simulink model "Wrist_Force_Control_v1_2"  (R2020a)
settings: Solver=ode4  StartTime=0.0  StopTime=inf  FixedStep=0.004  RelTol=1e-3  EnableMultiTasking=on
libraries: xpcethercatlib x17, slrtlib x12, simulink x4, simulink_extras x2
settings Model: xpc_rtwmakecfg_data=_xpcethercatlib_  SimulationMode=external  Creator=Ali  LastModifiedBy=Ali
settings SolverCC: ConcurrentTasks=on  AutoInsertRateTranBlk=on
settings DataIOCC: SaveFormat=StructureWithTime
settings OptimizationCC: BlockReduction=off  OptimizeBlockIOStorage=off
settings HardwareCC: ProdBitPerPointer=32  ProdBitPerSizeT=32  ProdBitPerPtrDiffT=32  ProdLargestAtomicFloat=None  ProdWordSize=32  ProdLongLongMode=on  ProdHWDeviceType=Generic->32-bit x86 compatible
settings RTWCC: Description=Simulink Real-Time  SystemTargetFile=slrt.tlc  TemplateMakefile=slrt_default_tmf  CodeExecutionProfiling=on  RTWCompilerOptimization=on
settings SimulinkRealTimeCC: SupportVariableSizeSignals=on  RL32LogTETModifier=off  xPCConcurrentTasks=on

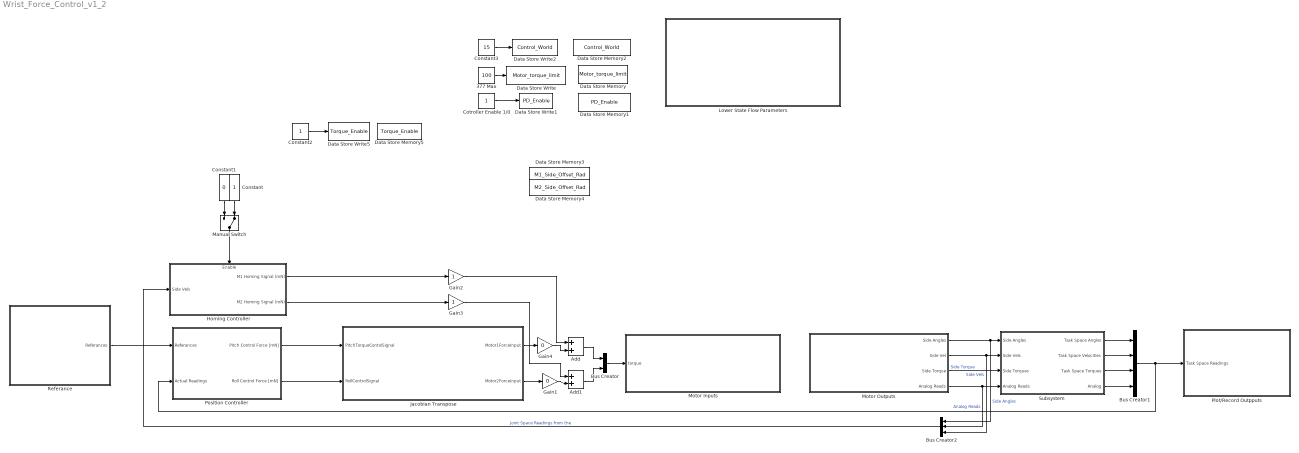
== system Wrist_Force_Control_v1_2 ==
  377 Max : Constant  Value=100
  Add : Sum
  Add1 : Sum
  Bus Creator : BusCreator  Inputs=2
  Bus Creator1 : BusCreator  Inputs=4
  Bus Creator2 : BusCreator  Inputs=3
  Constant : Constant
  Constant1 : Constant  Value=0
  Constant2 : Constant
  Constant3 : Constant  Value=15
  Cotroller Enable 1/0 : Constant
  Data Store Memory : DataStoreMemory  DataStoreName=Motor_torque_limit  ReadBeforeWriteMsg=warning  WriteAfterWriteMsg=warning  WriteAfterReadMsg=warning  ShowAdditionalParam=off
  Data Store Memory1 : DataStoreMemory  DataStoreName=PD_Enable  ReadBeforeWriteMsg=warning  WriteAfterWriteMsg=warning  WriteAfterReadMsg=warning  ShowAdditionalParam=off
  Data Store Memory2 : DataStoreMemory  DataStoreName=Control_World  ReadBeforeWriteMsg=warning  WriteAfterWriteMsg=warning  WriteAfterReadMsg=warning  ShowAdditionalParam=off
  Data Store Memory3 : DataStoreMemory  DataStoreName=M1_Side_Offset_Rad  ReadBeforeWriteMsg=warning  WriteAfterWriteMsg=warning  WriteAfterReadMsg=warning  ShowAdditionalParam=off
  Data Store Memory4 : DataStoreMemory  DataStoreName=M2_Side_Offset_Rad  ReadBeforeWriteMsg=warning  WriteAfterWriteMsg=warning  WriteAfterReadMsg=warning  ShowAdditionalParam=off
  Data Store Memory5 : DataStoreMemory  DataStoreName=Torque_Enable  ReadBeforeWriteMsg=warning  WriteAfterWriteMsg=warning  WriteAfterReadMsg=warning  ShowAdditionalParam=off
  Data Store Write : DataStoreWrite  DataStoreName=Motor_torque_limit
  Data Store Write1 : DataStoreWrite  DataStoreName=PD_Enable
  Data Store Write2 : DataStoreWrite  DataStoreName=Control_World
  Data Store Write5 : DataStoreWrite  DataStoreName=Torque_Enable
  Gain1 : Gain  Gain=0
  Gain2 : Gain
  Gain3 : Gain
  Gain4 : Gain  Gain=0
  Homing Controller : Subsystem
      settings: PortSchema="{\"entries\":[{\"content\":{\"sides\":[{\"content\":{\"connectorIds\":[\"In1\"]},\"type\":\"ConnectorPlacement.EquallySpacedRectSide\",\"uuid\":\"26584363-ec53-497c-894b-995f7264c9bf\"},{\"content\":{\"connectorIds\":[\"Out1\",\"Out2\"],\"side\":\"RIGHT\"},\"type\":\"ConnectorPlacement.EquallySpacedRectSide\",\"uuid\":\"844e0c8d-cb22-473f-a9ac-689e1ce20542\"},{\"content\":{\"connectorIds\":[\"In2\"],\"side\":\"TOP\"},\"type\":\"ConnectorPlacement.EquallySpacedRectSide\",\"uuid\":\"deb693f2-d5e7-4749-a5a4-0b0846583d72\"}]},\"type\":\"ConnectorPlacement.EquallySpacedConnector\",\"uuid\":\"b5658ea7-d246-475e-8f63-4337504fb7e8\"}],\"packageUris\":[\"http://schema.mathworks.com/mf0/Connector/19700101\"],\"version\":\"1.0\"}"
  Jacobian Transpose : MATLAB Function  TreatAsAtomicUnit=on
  Lower State Flow Parameters : Subsystem
  Manual Switch : ManualSwitch  CurrentSetting=0
  Motor Inputs : Subsystem
  Motor Outputs : Subsystem
  Plot/Record Outpputs : Subsystem
  Position Controller : Subsystem
  Referance : Subsystem
  Subsystem : Subsystem
  wires:
  Constant3/1 -> Data Store Write2/1
  377 Max/1 -> Data Store Write/1
  Bus Creator/1 -> Motor Inputs/1(torque)
  Motor Outputs/1(Side Angles) -> Bus Creator2/1, Subsystem/1(Side Angles)  "Side Angles"
  Motor Outputs/2(Side Vel) -> Bus Creator2/3, Subsystem/2(Side Vels)  "Side Vels"
  Motor Outputs/3(Side Torque) -> Subsystem/3(Side Torques)  "Side Torque"
  Motor Outputs/4(Analog Reads) -> Bus Creator2/2, Subsystem/4(Analog Reads)  "Analog Reads"
  Subsystem/1(Task Space Angles) -> Bus Creator1/1
  Subsystem/2(Task Space Velocities) -> Bus Creator1/2
  Subsystem/3(Task Space Torques) -> Bus Creator1/3
  Subsystem/4(Analog) -> Bus Creator1/4
  Bus Creator1/1 -> Position Controller/2(Actual Readings), Plot/Record Outpputs/1(Task Space Readings)
  Referance/1(Referances) -> Position Controller/1(Referances)
  Cotroller Enable 1/0/1 -> Data Store Write1/1
  Position Controller/1(Pitch Control Force [mN]) -> Jacobian Transpose/1(PitchTorqueContolSignal)
  Position Controller/2(Roll Control Force [mN]) -> Jacobian Transpose/2(RollControlSignal)
  Jacobian Transpose/1(Motor1ForceInput) -> Gain4/1
  Add/1 -> Bus Creator/1
  Jacobian Transpose/2(Motor2ForceInput) -> Gain1/1
  Add1/1 -> Bus Creator/2
  Constant/1 -> Manual Switch/2
  Constant1/1 -> Manual Switch/1
  Constant2/1 -> Data Store Write5/1
  Gain4/1 -> Add/2
  Gain1/1 -> Add1/2
  Gain2/1 -> Add/1
  Gain3/1 -> Add1/1
  Manual Switch/1 -> Homing Controller/2(Enable)
  Homing Controller/1(M1 Homing Signal (mN)) -> Gain2/1
  Homing Controller/2(M2 Homing Signal (mN)) -> Gain3/1
  Bus Creator2/1 -> Homing Controller/1(Side Vels)  "Joint Space Readings from the"

== system Wrist_Force_Control_v1_2/Homing Controller ==
  Side Vels : Inport
  Enable : Inport  Port=2
  Analog Homing Controllers : Subsystem
  Bus Selector : BusSelector  OutputSignals=Analog Reads,Side Vels,Side Angles
  Clock : Subsystem
  M1 Homing Signal (mN) : Outport
  M2 Homing Signal (mN) : Outport  Port=2
  wires:
  Analog Homing Controllers/1(M1 Homing Signal) -> M1 Homing Signal (mN)/1  "M1 Homing Signal (mN)"
  Clock/1(Enabling Signal) -> Analog Homing Controllers/Enable
  Enable/1 -> Clock/Enable
  Analog Homing Controllers/2(M2 Homing Signal) -> M2 Homing Signal (mN)/1  "M2 Homing Signal (mN)"
  Side Vels/1 -> Bus Selector/1
  Bus Selector/1 -> Analog Homing Controllers/1(Analog Signals)  "<Analog Reads>"
  Bus Selector/2 -> Analog Homing Controllers/2(Side Vels)  "<Side Vels>"
  Bus Selector/3 -> Analog Homing Controllers/3(Side Angles)  "<Side Angles>"

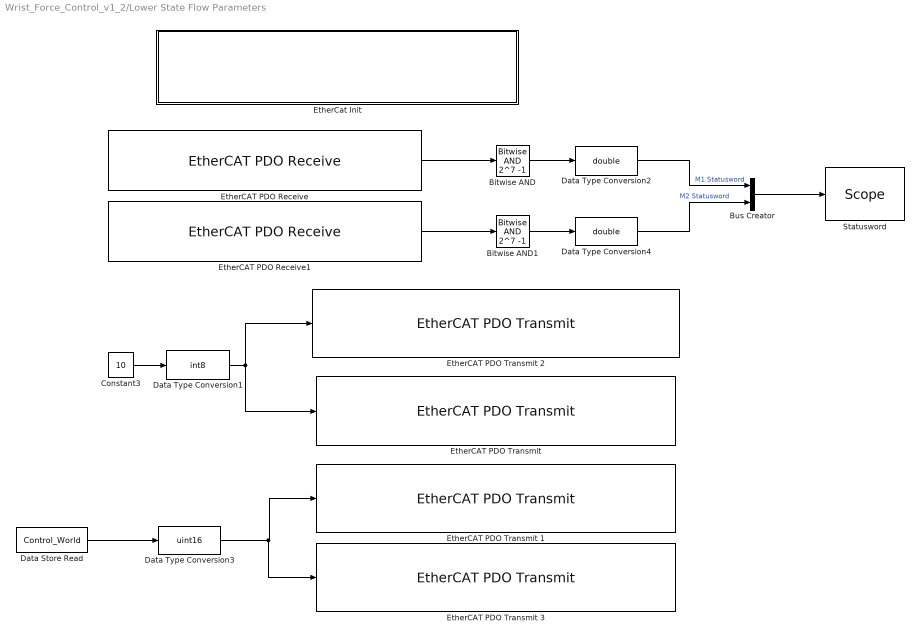
== system Wrist_Force_Control_v1_2/Lower State Flow Parameters ==
  Bitwise AND : simulink/Logic and Bit Operations/Bitwise Operator  logicop=AND  UseBitMask=on  BitMask=2^7 -1  BitMaskRealWorld=Stored Integer
  Bitwise AND1 : simulink/Logic and Bit Operations/Bitwise Operator  logicop=AND  UseBitMask=on  BitMask=2^7 -1  BitMaskRealWorld=Stored Integer
  Bus Creator : BusCreator  Inputs=2
  Constant3 : Constant  Value=10
  Data Store Read : DataStoreRead  DataStoreName=Control_World
  Data Type Conversion1 : DataTypeConversion  OutDataTypeStr=int8
  Data Type Conversion2 : DataTypeConversion  OutDataTypeStr=double
  Data Type Conversion3 : DataTypeConversion  OutDataTypeStr=uint16
  Data Type Conversion4 : DataTypeConversion  OutDataTypeStr=double
  EtherCAT PDO Receive : xpcethercatlib/EtherCAT PDO Receive  Priority=2  sig_name=M1.Module 1 (CST Mode).CST Inputs.Statusword  sig_offset=568  sig_type=uint16  type_size=16  sig_dim=1  device_id=0  sample_time=0.004000
      settings: SourceProductBaseCode=XP
  EtherCAT PDO Receive1 : xpcethercatlib/EtherCAT PDO Receive  Priority=2  sig_name=M2.Module 1 (CST Mode).CST Inputs.Statusword  sig_offset=696  sig_type=uint16  type_size=16  sig_dim=1  device_id=0  sample_time=0.004000
      settings: SourceProductBaseCode=XP
  "EtherCAT PDO Transmit " : xpcethercatlib/EtherCAT PDO Transmit   Priority=3  sig_name=M2.Module 1 (CST Mode).CST Outputs.Mode of operation  sig_offset=728  sig_type=int8  type_size=8  sig_dim=1  device_id=0  sample_time=0.004000
      settings: SourceProductBaseCode=XP
  EtherCAT PDO Transmit 1 : xpcethercatlib/EtherCAT PDO Transmit   Priority=3  sig_name=M1.Module 1 (CST Mode).CST Outputs.Controlword  sig_offset=568  sig_type=uint16  type_size=16  sig_dim=1  device_id=0  sample_time=0.004000
      settings: SourceProductBaseCode=XP
  EtherCAT PDO Transmit 2 : xpcethercatlib/EtherCAT PDO Transmit   Priority=3  sig_name=M1.Module 1 (CST Mode).CST Outputs.Mode of operation  sig_offset=600  sig_type=int8  type_size=8  sig_dim=1  device_id=0  sample_time=0.004000
      settings: SourceProductBaseCode=XP
  EtherCAT PDO Transmit 3 : xpcethercatlib/EtherCAT PDO Transmit   Priority=3  sig_name=M2.Module 1 (CST Mode).CST Outputs.Controlword  sig_offset=696  sig_type=uint16  type_size=16  sig_dim=1  device_id=0  sample_time=0.004000
      settings: SourceProductBaseCode=XP
  EtherCat Init : Subsystem
  Statusword : slrtlib/Displays and Logging/Scope   scopeno=1  scopetype=Target  autostart=on  viewmode=Numerical  formatstr='%15.6f'  grid=on  ylimits=[0,0]  nosamples=100  noprepostsamples=0  interleave=5  triggermode=FreeRun  triggersignal=1  trigsignalfromport=off  triggerlevel=0.0  triggerslope=Either  triggerscope=1  triggersample=0  filename=data.dat  mode=Lazy  writesize=512  autorestart=off  dynamicfilemode=off  maxwritefilesize=512*1024^2
  wires:
  Bitwise AND/1 -> Data Type Conversion2/1
  EtherCAT PDO Receive/1 -> Bitwise AND/1
  Data Store Read/1 -> Data Type Conversion3/1
  Constant3/1 -> Data Type Conversion1/1
  Data Type Conversion1/1 -> EtherCAT PDO Transmit 2/1, "EtherCAT PDO Transmit "/1
  Bitwise AND1/1 -> Data Type Conversion4/1
  EtherCAT PDO Receive1/1 -> Bitwise AND1/1
  Data Type Conversion4/1 -> Bus Creator/2  "M2 Statusword"
  Bus Creator/1 -> Statusword/1
  Data Type Conversion2/1 -> Bus Creator/1  "M1 Statusword"
  Data Type Conversion3/1 -> EtherCAT PDO Transmit 3/1, EtherCAT PDO Transmit 1/1

== system Wrist_Force_Control_v1_2/Motor Inputs ==
  torque : Inport
  "M1 Target Torque " : xpcethercatlib/EtherCAT PDO Transmit   Priority=3  sig_name=M1.Module 1 (CST Mode).CST Outputs.Target torque  sig_offset=584  sig_type=int16  type_size=16  sig_dim=1  device_id=0  sample_time=0.004000
      settings: SourceProductBaseCode=XP
  M2 Target Torque : xpcethercatlib/EtherCAT PDO Transmit   Priority=3  sig_name=M2.Module 1 (CST Mode).CST Outputs.Target torque  sig_offset=712  sig_type=int16  type_size=16  sig_dim=1  device_id=0  sample_time=0.004000
      settings: SourceProductBaseCode=XP
  "Scope " : slrtlib/Displays and Logging/Scope   Commented=on  scopeno=2  scopetype=Target  autostart=on  viewmode=Graphical rolling  formatstr='%15.6f'  grid=on  ylimits=[0,0]  nosamples=100  noprepostsamples=0  interleave=5  triggermode=FreeRun  triggersignal=1  trigsignalfromport=off  triggerlevel=0.0  triggerslope=Either  triggerscope=1  triggersample=0  filename=data.dat  mode=Lazy  writesize=512  autorestart=off  dynamicfilemode=off  maxwritefilesize=512*1024^2
  "Torque Mappig and Saturation " : Subsystem
  wires:
  torque/1 -> "Torque Mappig and Saturation "/1(torque)
  "Torque Mappig and Saturation "/3(Motor Torques) -> "Scope "/1
  "Torque Mappig and Saturation "/1(M1_torque) -> "M1 Target Torque "/1
  "Torque Mappig and Saturation "/2(M2_torque) -> M2 Target Torque/1

== system Wrist_Force_Control_v1_2/Motor Outputs ==
  Analog Readigs : Subsystem
  Angle Readigs : Subsystem
  Bus Creator : BusCreator  Inputs=2
  Torque Readings : Subsystem
  Velocity Readings : Subsystem
  Side Angles : Outport
  Side Vel : Outport  Port=2
  Side Torque : Outport  Port=3
  Analog Reads : Outport  Port=4
  wires:
  Velocity Readings/1(Side Vel) -> Side Vel/1
  Torque Readings/1(Side Torque) -> Side Torque/1
  Angle Readigs/1(Side angles) -> Side Angles/1
  Analog Readigs/1(M1 Analog Reads (mV)) -> Bus Creator/1  "M1 Analog Reads"
  Analog Readigs/2(M2 Analog Reads (mV)) -> Bus Creator/2  "M2 Analog Reads"
  Bus Creator/1 -> Analog Reads/1

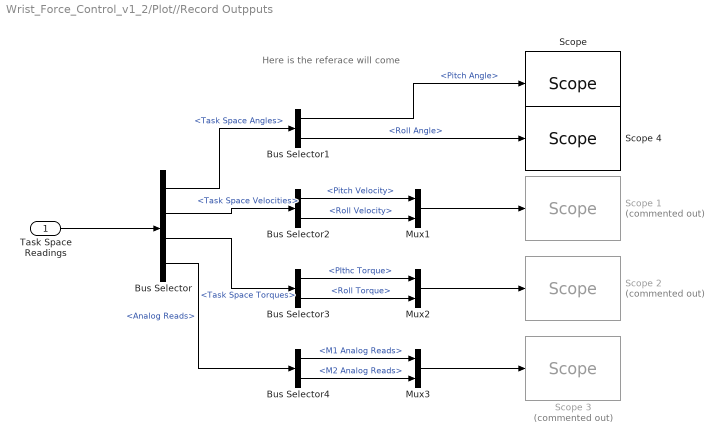
== system Wrist_Force_Control_v1_2/Plot//Record Outpputs ==
  note: Here is the referace will come
  Task Space Readings : Inport
  Bus Selector : BusSelector  OutputSignals=Task Space Angles,Task Space Velocities,Task Space Torques,Analog Reads
  Bus Selector1 : BusSelector  OutputSignals=Pitch Angle,Roll Angle
  Bus Selector2 : BusSelector  OutputSignals=Pitch Velocity,Roll Velocity
  Bus Selector3 : BusSelector  OutputSignals=PIthc Torque,Roll Torque
  Bus Selector4 : BusSelector  OutputSignals=M1 Analog Reads,M2 Analog Reads
  Mux1 : Mux  Inputs=2
  Mux2 : Mux  Inputs=2
  Mux3 : Mux  Inputs=2
  "Scope " : slrtlib/Displays and Logging/Scope   scopeno=8  scopetype=Target  autostart=on  viewmode=Graphical rolling  formatstr='%15.6f'  grid=on  ylimits=[0,0]  nosamples=100  noprepostsamples=0  interleave=5  triggermode=FreeRun  triggersignal=1  trigsignalfromport=off  triggerlevel=0.0  triggerslope=Either  triggerscope=1  triggersample=0  filename=data.dat  mode=Lazy  writesize=512  autorestart=off  dynamicfilemode=off  maxwritefilesize=512*1024^2
  Scope 1 : slrtlib/Displays and Logging/Scope   Commented=on  scopeno=4  scopetype=Target  autostart=on  viewmode=Graphical rolling  formatstr='%15.6f'  grid=on  ylimits=[0,0]  nosamples=500  noprepostsamples=0  interleave=20  triggermode=FreeRun  triggersignal=1  trigsignalfromport=off  triggerlevel=0.0  triggerslope=Either  triggerscope=1  triggersample=0  filename=data.dat  mode=Lazy  writesize=512  autorestart=off  dynamicfilemode=off  maxwritefilesize=512*1024^2
  Scope 2 : slrtlib/Displays and Logging/Scope   Commented=on  scopeno=5  scopetype=Target  autostart=on  viewmode=Graphical rolling  formatstr='%15.6f'  grid=on  ylimits=[0,0]  nosamples=500  noprepostsamples=0  interleave=20  triggermode=FreeRun  triggersignal=1  trigsignalfromport=off  triggerlevel=0.0  triggerslope=Either  triggerscope=1  triggersample=0  filename=data.dat  mode=Lazy  writesize=512  autorestart=off  dynamicfilemode=off  maxwritefilesize=512*1024^2
  Scope 3 : slrtlib/Displays and Logging/Scope   Commented=on  scopeno=6  scopetype=Target  autostart=on  viewmode=Graphical rolling  formatstr='%15.6f'  grid=on  ylimits=[0,0]  nosamples=500  noprepostsamples=0  interleave=20  triggermode=FreeRun  triggersignal=1  trigsignalfromport=off  triggerlevel=0.0  triggerslope=Either  triggerscope=1  triggersample=0  filename=data.dat  mode=Lazy  writesize=512  autorestart=off  dynamicfilemode=off  maxwritefilesize=512*1024^2
  Scope 4 : slrtlib/Displays and Logging/Scope   scopeno=9  scopetype=Target  autostart=on  viewmode=Graphical rolling  formatstr='%15.6f'  grid=on  ylimits=[0,0]  nosamples=100  noprepostsamples=0  interleave=5  triggermode=FreeRun  triggersignal=1  trigsignalfromport=off  triggerlevel=0.0  triggerslope=Either  triggerscope=1  triggersample=0  filename=data.dat  mode=Lazy  writesize=512  autorestart=off  dynamicfilemode=off  maxwritefilesize=512*1024^2
  wires:
  Task Space Readings/1 -> Bus Selector/1
  Bus Selector/1 -> Bus Selector1/1  "<Task Space Angles>"
  Bus Selector1/1 -> "Scope "/1  "<Pitch Angle>"
  Bus Selector1/2 -> Scope 4/1  "<Roll Angle>"
  Bus Selector2/1 -> Mux1/1  "<Pitch Velocity>"
  Mux1/1 -> Scope 1/1
  Bus Selector2/2 -> Mux1/2  "<Roll Velocity>"
  Bus Selector/2 -> Bus Selector2/1  "<Task Space Velocities>"
  Bus Selector3/2 -> Mux2/2  "<Roll Torque>"
  Bus Selector3/1 -> Mux2/1  "<PIthc Torque>"
  Mux2/1 -> Scope 2/1
  Bus Selector/3 -> Bus Selector3/1  "<Task Space Torques>"
  Mux3/1 -> Scope 3/1
  Bus Selector4/2 -> Mux3/2  "<M2 Analog Reads>"
  Bus Selector4/1 -> Mux3/1  "<M1 Analog Reads>"
  Bus Selector/4 -> Bus Selector4/1  "<Analog Reads>"

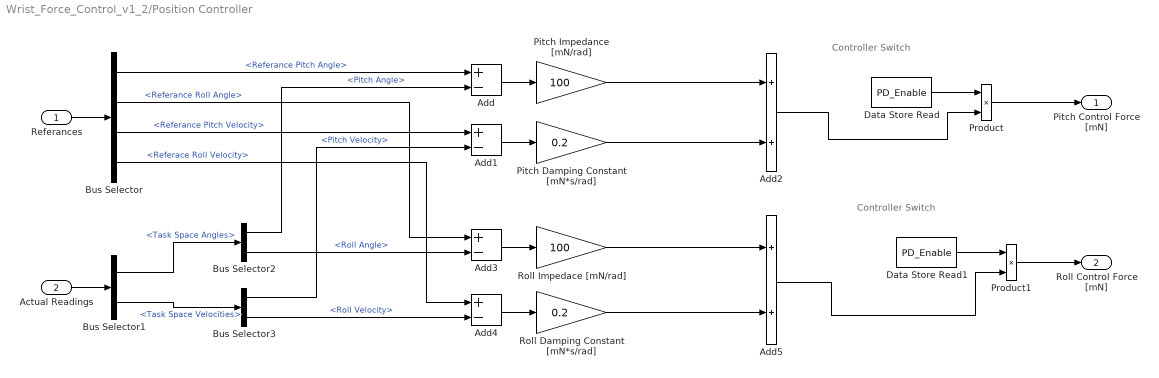
== system Wrist_Force_Control_v1_2/Position Controller ==
  note: Controller Switch
  note: Controller Switch
  Referances : Inport
  Actual Readings : Inport  Port=2
  Add{,1,3..4} (4 alike) : Sum  Inputs=+-
  Add2 : Sum
  Add5 : Sum
  Bus Selector : BusSelector  OutputSignals=Referance Pitch Angle,Referance Roll Angle,Referance Pitch Velocity,Referace Roll Velocity
  Bus Selector1 : BusSelector  OutputSignals=Task Space Angles,Task Space Velocities
  Bus Selector2 : BusSelector  OutputSignals=Pitch Angle,Roll Angle
  Bus Selector3 : BusSelector  OutputSignals=Pitch Velocity,Roll Velocity
  Data Store Read : DataStoreRead  DataStoreName=PD_Enable
  Data Store Read1 : DataStoreRead  DataStoreName=PD_Enable
  Pitch Damping Constant [mN*s/rad] : Gain  Gain=0.2
  Pitch Impedance [mN/rad] : Gain  Gain=100
  Product : Product
  Product1 : Product
  Roll Damping Constant [mN*s/rad] : Gain  Gain=0.2
  Roll Impedace [mN/rad] : Gain  Gain=100
  Pitch Control Force [mN] : Outport
  Roll Control Force [mN] : Outport  Port=2
  wires:
  Referances/1 -> Bus Selector/1
  Bus Selector/1 -> Add/1  "<Referance Pitch Angle>"
  Bus Selector/2 -> Add3/1  "<Referance Roll Angle>"
  Bus Selector/4 -> Add4/1  "<Referace Roll Velocity>"
  Actual Readings/1 -> Bus Selector1/1
  Add/1 -> Pitch Impedance [mN/rad]/1
  Pitch Damping Constant [mN*s/rad]/1 -> Add2/2
  Product/1 -> Pitch Control Force [mN]/1
  Add2/1 -> Product/2
  Data Store Read/1 -> Product/1
  Add1/1 -> Pitch Damping Constant [mN*s/rad]/1
  Bus Selector1/1 -> Bus Selector2/1  "<Task Space Angles>"
  Bus Selector1/2 -> Bus Selector3/1  "<Task Space Velocities>"
  Bus Selector2/1 -> Add/2  "<Pitch Angle>"
  Bus Selector/3 -> Add1/1  "<Referance Pitch Velocity>"
  Bus Selector3/1 -> Add1/2  "<Pitch Velocity>"
  Bus Selector3/2 -> Add4/2  "<Roll Velocity>"
  Bus Selector2/2 -> Add3/2  "<Roll Angle>"
  Add3/1 -> Roll Impedace [mN/rad]/1
  Add4/1 -> Roll Damping Constant [mN*s/rad]/1
  Pitch Impedance [mN/rad]/1 -> Add2/1
  Roll Impedace [mN/rad]/1 -> Add5/1
  Roll Damping Constant [mN*s/rad]/1 -> Add5/2
  Product1/1 -> Roll Control Force [mN]/1
  Add5/1 -> Product1/2
  Data Store Read1/1 -> Product1/1

== system Wrist_Force_Control_v1_2/Referance ==
  Bus Creator : BusCreator  Inputs=4
  Degrees to Radians : simulink_extras/Transformations/Degrees to Radians
  Degrees to Radians1 : simulink_extras/Transformations/Degrees to Radians
  Pitch Degree : Constant
  Pitch Velocity (rad/s) : Constant
  Roll Degree : Constant
  Roll Velocity (rad/s) : Constant
  Referances : Outport
  wires:
  Pitch Degree/1 -> Degrees to Radians/1
  Roll Degree/1 -> Degrees to Radians1/1
  Degrees to Radians1/1 -> Bus Creator/2  "Referance Roll Angle"
  Pitch Velocity (rad/s)/1 -> Bus Creator/3  "Referance Pitch Velocity"
  Roll Velocity (rad/s)/1 -> Bus Creator/4  "Referace Roll Velocity"
  Degrees to Radians/1 -> Bus Creator/1  "Referance Pitch Angle"
  Bus Creator/1 -> Referances/1

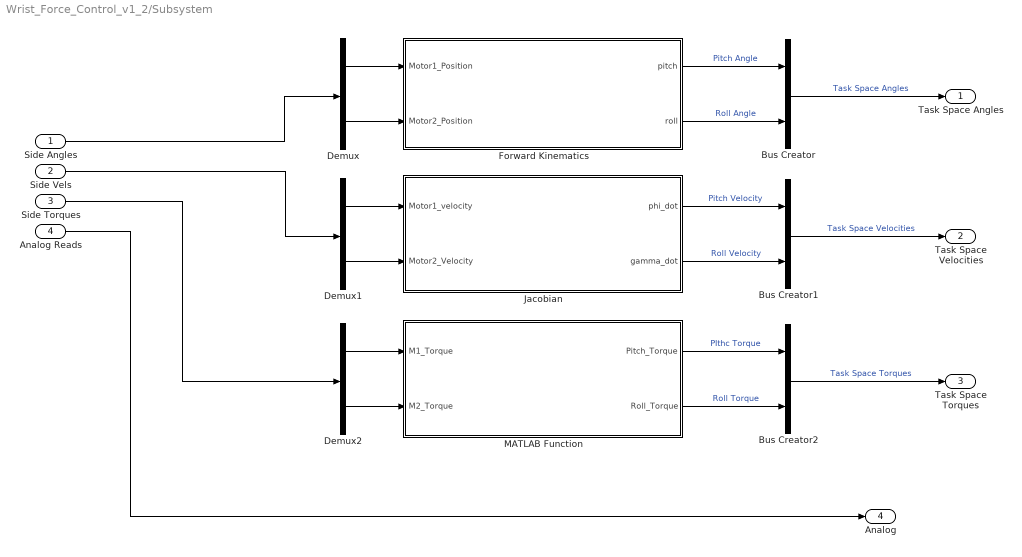
== system Wrist_Force_Control_v1_2/Subsystem ==
  Side Angles : Inport
  Side Vels : Inport  Port=2
  Side Torques : Inport  Port=3
  Analog Reads : Inport  Port=4
  Bus Creator : BusCreator  Inputs=2
  Bus Creator1 : BusCreator  Inputs=2
  Bus Creator2 : BusCreator  Inputs=2
  Demux : Demux  Outputs=2
  Demux1 : Demux  Outputs=2
  Demux2 : Demux  Outputs=2
  Forward Kinematics : MATLAB Function  TreatAsAtomicUnit=on
  Jacobian : MATLAB Function  TreatAsAtomicUnit=on
  MATLAB Function : MATLAB Function  TreatAsAtomicUnit=on
  Task Space Angles : Outport
  Task Space Velocities : Outport  Port=2
  Task Space Torques : Outport  Port=3
  Analog : Outport  Port=4
  wires:
  Analog Reads/1 -> Analog/1
  Side Torques/1 -> Demux2/1
  Side Angles/1 -> Demux/1
  Demux/1 -> Forward Kinematics/1(Motor1_Position)
  Demux/2 -> Forward Kinematics/2(Motor2_Position)
  Demux1/2 -> Jacobian/2(Motor2_Velocity)
  Demux1/1 -> Jacobian/1(Motor1_velocity)
  Side Vels/1 -> Demux1/1
  Jacobian/1(phi_dot) -> Bus Creator1/1  "Pitch Velocity"
  Jacobian/2(gamma_dot) -> Bus Creator1/2  "Roll Velocity"
  Demux2/1 -> MATLAB Function/1(M1_Torque)
  Demux2/2 -> MATLAB Function/2(M2_Torque)
  Forward Kinematics/1(pitch) -> Bus Creator/1  "Pitch Angle"
  Forward Kinematics/2(roll) -> Bus Creator/2  "Roll Angle"
  Bus Creator/1 -> Task Space Angles/1  "Task Space Angles"
  MATLAB Function/1(Pitch_Torque) -> Bus Creator2/1  "PIthc Torque"
  MATLAB Function/2(Roll_Torque) -> Bus Creator2/2  "Roll Torque"
  Bus Creator2/1 -> Task Space Torques/1  "Task Space Torques"
  Bus Creator1/1 -> Task Space Velocities/1  "Task Space Velocities"

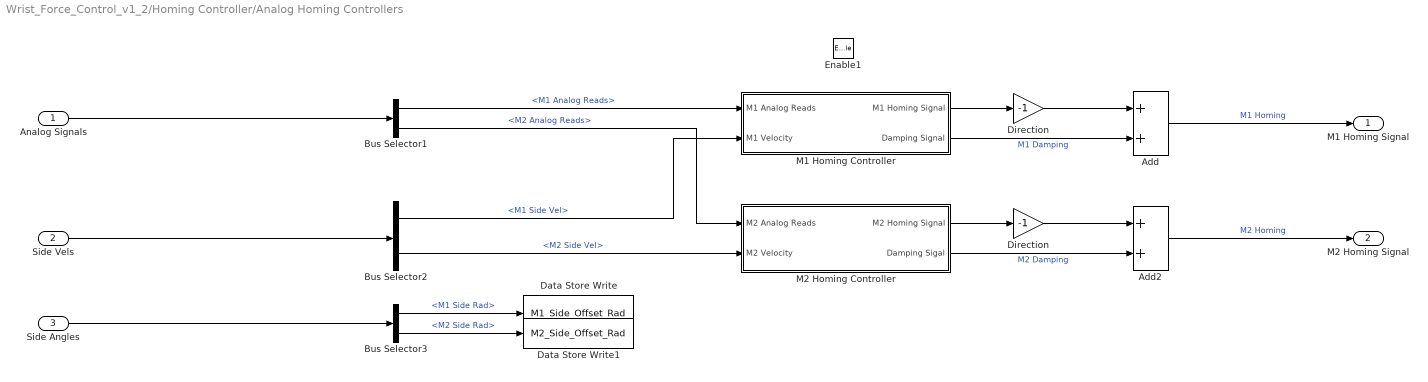
== system Wrist_Force_Control_v1_2/Homing Controller/Analog Homing Controllers ==
  Analog Signals : Inport
  Side Vels : Inport  Port=2
  Side Angles : Inport  Port=3
  Enable1 : EnablePort
  Add : Sum
  Add2 : Sum
  Bus Selector1 : BusSelector  OutputSignals=M1 Analog Reads,M2 Analog Reads
  Bus Selector2 : BusSelector  OutputSignals=M1 Side Vel,M2 Side Vel
  Bus Selector3 : BusSelector  OutputSignals=M1 Side Rad,M2 Side Rad
  Data Store Write : DataStoreWrite  DataStoreName=M1_Side_Offset_Rad
  Data Store Write1 : DataStoreWrite  DataStoreName=M2_Side_Offset_Rad
  Direction : Gain  Gain=-1
  "Direction " : Gain  Gain=-1
  M1 Homing Controller : Subsystem
  M2 Homing Controller : Subsystem
  M1 Homing Signal : Outport
  M2 Homing Signal : Outport  Port=2
  wires:
  Bus Selector1/1 -> M1 Homing Controller/1(M1 Analog Reads)  "<M1 Analog Reads>"
  Analog Signals/1 -> Bus Selector1/1
  Bus Selector1/2 -> M2 Homing Controller/1(M2 Analog Reads)  "<M2 Analog Reads>"
  M1 Homing Controller/1(M1 Homing Signal) -> Direction/1
  M2 Homing Controller/1(M2 Homing Signal) -> "Direction "/1
  Side Vels/1 -> Bus Selector2/1
  Direction/1 -> Add/1
  M1 Homing Controller/2(Damping Signal) -> Add/2  "M1 Damping"
  Add/1 -> M1 Homing Signal/1  "M1 Homing"
  Add2/1 -> M2 Homing Signal/1  "M2 Homing"
  "Direction "/1 -> Add2/1
  M2 Homing Controller/2(Damping Sigal) -> Add2/2  "M2 Damping"
  Bus Selector2/1 -> M1 Homing Controller/2(M1 Velocity)  "<M1 Side Vel>"
  Bus Selector2/2 -> M2 Homing Controller/2(M2 Velocity)  "<M2 Side Vel>"
  Side Angles/1 -> Bus Selector3/1
  Bus Selector3/1 -> Data Store Write/1  "<M1 Side Rad>"
  Bus Selector3/2 -> Data Store Write1/1  "<M2 Side Rad>"

== system Wrist_Force_Control_v1_2/Homing Controller/Clock ==
  Enable : EnablePort
  Clock : Clock
  Constant5 : Constant  Value=10
  Relational Operator : RelationalOperator  OutDataTypeStr=boolean  RndMeth=Simplest
  Enabling Signal : Outport
  wires:
  Clock/1 -> Relational Operator/1
  Constant5/1 -> Relational Operator/2
  Relational Operator/1 -> Enabling Signal/1

== system Wrist_Force_Control_v1_2/Lower State Flow Parameters/EtherCat Init ==
  "EtherCAT Init " : xpcethercatlib/EtherCAT Init   Priority=0  config_file=C:\Users\Ali\Desktop\Wrist_Control_Test\XML_Config_File\Force_Control_v2.5_250Hz.xml  device_id=0  pci_bus=2  pci_slot=0  pci_function=0  initstate=2  dctuning=0  enaDebug=off  enaDC=on  errLink=off  masterDbg=off  stateChgDbg=off  baseClock=off  masterCfg=off  logFile='c:\dbglog.txt'  sample_time=0.004000  DCMode=2
      settings: SourceProductBaseCode=XP
  Terminator : Terminator
  wires:
  "EtherCAT Init "/1 -> Terminator/1

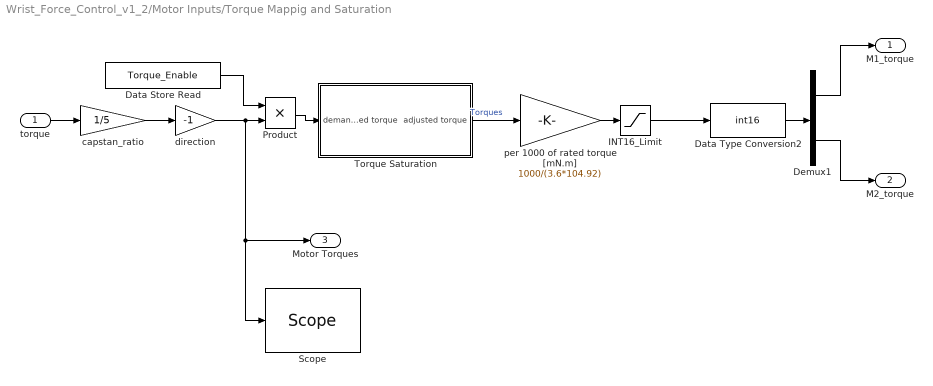
== system Wrist_Force_Control_v1_2/Motor Inputs/Torque Mappig and Saturation  ==
  torque : Inport
  Data Store Read : DataStoreRead  DataStoreName=Torque_Enable
  Data Type Conversion2 : DataTypeConversion  OutDataTypeStr=int16
  Demux1 : Demux  Outputs=2
  INT16_Limit : Saturate  UpperLimit=[2^15-1 2^15-1]  LowerLimit=[-2^15 -2^15]
  Product : Product
  "Scope " : slrtlib/Displays and Logging/Scope   scopeno=5  scopetype=Target  autostart=on  viewmode=Numerical  formatstr='%15.6f'  grid=on  ylimits=[0,0]  nosamples=100  noprepostsamples=0  interleave=5  triggermode=FreeRun  triggersignal=1  trigsignalfromport=off  triggerlevel=0.0  triggerslope=Either  triggerscope=1  triggersample=0  filename=data.dat  mode=Lazy  writesize=512  autorestart=off  dynamicfilemode=off  maxwritefilesize=512*1024^2
  Torque Saturation : Subsystem
  capstan_ratio : Gain  Gain=1/5
  direction : Gain  Gain=-1  OutDataTypeStr=double
  per 1000 of rated torque [mN.m] : Gain  Gain=1000/(3.6*104.92)  OutDataTypeStr=double
  M1_torque : Outport  VectorParamsAs1DForOutWhenUnconnected=off
  M2_torque : Outport  Port=2  VectorParamsAs1DForOutWhenUnconnected=off
  Motor Torques : Outport  Port=3
  wires:
  direction/1 -> Product/2, "Scope "/1, Motor Torques/1
  Demux1/1 -> M1_torque/1
  Demux1/2 -> M2_torque/1
  per 1000 of rated torque [mN.m]/1 -> INT16_Limit/1
  Torque Saturation/1(adjusted torque) -> per 1000 of rated torque [mN.m]/1  "Torques"
  capstan_ratio/1 -> direction/1
  INT16_Limit/1 -> Data Type Conversion2/1
  torque/1 -> capstan_ratio/1
  Data Type Conversion2/1 -> Demux1/1
  Product/1 -> Torque Saturation/1(demanded torque)
  Data Store Read/1 -> Product/1

== system Wrist_Force_Control_v1_2/Motor Outputs/Analog Readigs ==
  Cast To Double : DataTypeConversion  OutDataTypeStr=double
  Cast To Double1 : DataTypeConversion  OutDataTypeStr=double
  EtherCAT PDO Receive : xpcethercatlib/EtherCAT PDO Receive  Priority=2  sig_name=M1.Module 1 (CST Mode).CST Inputs.Analog input general purpose A  sig_offset=680  sig_type=int16  type_size=16  sig_dim=1  device_id=0  sample_time=0.004000
      settings: SourceProductBaseCode=XP
  EtherCAT PDO Receive1 : xpcethercatlib/EtherCAT PDO Receive  Priority=2  sig_name=M2.Module 1 (CST Mode).CST Inputs.Analog input general purpose A  sig_offset=808  sig_type=int16  type_size=16  sig_dim=1  device_id=0  sample_time=0.004000
      settings: SourceProductBaseCode=XP
  Scope 2 : slrtlib/Displays and Logging/Scope   scopeno=3  scopetype=Target  autostart=on  viewmode=Graphical rolling  formatstr='%15.6f'  grid=on  ylimits=[0,0]  nosamples=250  noprepostsamples=0  interleave=5  triggermode=FreeRun  triggersignal=1  trigsignalfromport=off  triggerlevel=0.0  triggerslope=Either  triggerscope=1  triggersample=0  filename=data.dat  mode=Lazy  writesize=512  autorestart=off  dynamicfilemode=off  maxwritefilesize=512*1024^2
  Scope 3 : slrtlib/Displays and Logging/Scope   scopeno=4  scopetype=Target  autostart=on  viewmode=Graphical rolling  formatstr='%15.6f'  grid=on  ylimits=[0,0]  nosamples=250  noprepostsamples=0  interleave=5  triggermode=FreeRun  triggersignal=1  trigsignalfromport=off  triggerlevel=0.0  triggerslope=Either  triggerscope=1  triggersample=0  filename=data.dat  mode=Lazy  writesize=512  autorestart=off  dynamicfilemode=off  maxwritefilesize=512*1024^2
  mV to count : Gain  Gain=1/10
  mV to count1 : Gain  Gain=1/10
  M1 Analog Reads (mV) : Outport
  M2 Analog Reads (mV) : Outport  Port=2
  wires:
  EtherCAT PDO Receive1/1 -> Cast To Double1/1
  EtherCAT PDO Receive/1 -> Cast To Double/1
  Cast To Double/1 -> mV to count1/1  "M1 Analog Read"
  Cast To Double1/1 -> mV to count/1  "M2 Analog Read"
  mV to count1/1 -> Scope 2/1, M1 Analog Reads (mV)/1  "M1 Analog Read"
  mV to count/1 -> Scope 3/1, M2 Analog Reads (mV)/1  "M2 Analog Read"

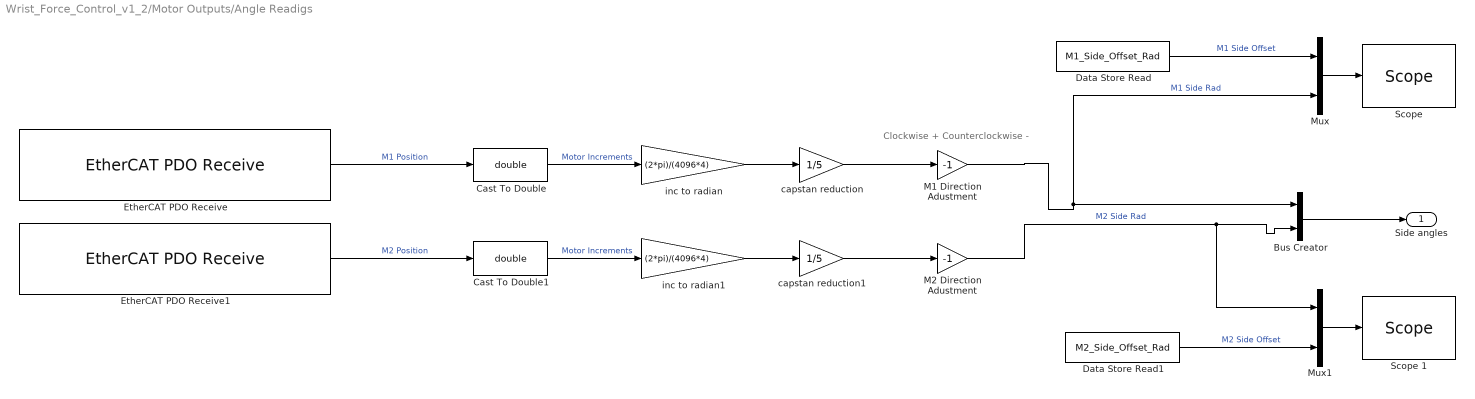
== system Wrist_Force_Control_v1_2/Motor Outputs/Angle Readigs ==
  note: Clockwise + Counterclockwise -
  Bus Creator : BusCreator  Inputs=2
  Cast To Double : DataTypeConversion  OutDataTypeStr=double
  Cast To Double1 : DataTypeConversion  OutDataTypeStr=double
  Data Store Read : DataStoreRead  DataStoreName=M1_Side_Offset_Rad
  Data Store Read1 : DataStoreRead  DataStoreName=M2_Side_Offset_Rad
  EtherCAT PDO Receive : xpcethercatlib/EtherCAT PDO Receive  Priority=2  sig_name=M1.Module 1 (CST Mode).CST Inputs.Position actual value  sig_offset=584  sig_type=int32  type_size=32  sig_dim=1  device_id=0  sample_time=0.004000
      settings: SourceProductBaseCode=XP
  EtherCAT PDO Receive1 : xpcethercatlib/EtherCAT PDO Receive  Priority=2  sig_name=M2.Module 1 (CST Mode).CST Inputs.Position actual value  sig_offset=712  sig_type=int32  type_size=32  sig_dim=1  device_id=0  sample_time=0.004000
      settings: SourceProductBaseCode=XP
  "M1 Direction Adustment " : Gain  Gain=-1
  M2 Direction Adustment : Gain  Gain=-1
  Mux : Mux  Inputs=2
  Mux1 : Mux  Inputs=2
  "Scope " : slrtlib/Displays and Logging/Scope   scopeno=2  scopetype=Target  autostart=on  viewmode=Numerical  formatstr='%15.6f'  grid=on  ylimits=[0,0]  nosamples=100  noprepostsamples=0  interleave=5  triggermode=FreeRun  triggersignal=1  trigsignalfromport=off  triggerlevel=0.0  triggerslope=Either  triggerscope=1  triggersample=0  filename=data.dat  mode=Lazy  writesize=512  autorestart=off  dynamicfilemode=off  maxwritefilesize=512*1024^2
  Scope 1 : slrtlib/Displays and Logging/Scope   scopeno=7  scopetype=Target  autostart=on  viewmode=Numerical  formatstr='%15.6f'  grid=on  ylimits=[0,0]  nosamples=100  noprepostsamples=0  interleave=5  triggermode=FreeRun  triggersignal=1  trigsignalfromport=off  triggerlevel=0.0  triggerslope=Either  triggerscope=1  triggersample=0  filename=data.dat  mode=Lazy  writesize=512  autorestart=off  dynamicfilemode=off  maxwritefilesize=512*1024^2
  capstan reduction : Gain  Gain=1/5
  capstan reduction1 : Gain  Gain=1/5
  inc to radian : Gain  Gain=(2*pi)/(4096*4)
  inc to radian1 : Gain  Gain=(2*pi)/(4096*4)
  Side angles : Outport
  wires:
  EtherCAT PDO Receive/1 -> Cast To Double/1  "M1 Position"
  Cast To Double/1 -> inc to radian/1  "Motor Increments"
  EtherCAT PDO Receive1/1 -> Cast To Double1/1  "M2 Position"
  inc to radian/1 -> capstan reduction/1
  capstan reduction/1 -> "M1 Direction Adustment "/1
  inc to radian1/1 -> capstan reduction1/1
  capstan reduction1/1 -> M2 Direction Adustment/1
  Cast To Double1/1 -> inc to radian1/1  "Motor Increments"
  "M1 Direction Adustment "/1 -> Bus Creator/1, Mux/2  "M1 Side Rad"
  Data Store Read/1 -> Mux/1  "M1 Side Offset"
  M2 Direction Adustment/1 -> Bus Creator/2, Mux1/1  "M2 Side Rad"
  Data Store Read1/1 -> Mux1/2  "M2 Side Offset"
  Mux/1 -> "Scope "/1
  Mux1/1 -> Scope 1/1
  Bus Creator/1 -> Side angles/1

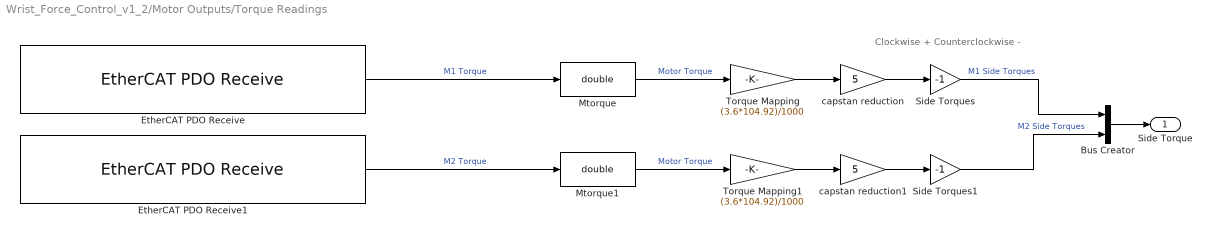
== system Wrist_Force_Control_v1_2/Motor Outputs/Torque Readings ==
  note: Clockwise + Counterclockwise -
  Bus Creator : BusCreator  Inputs=2
  EtherCAT PDO Receive : xpcethercatlib/EtherCAT PDO Receive  Priority=2  sig_name=M1.Module 1 (CST Mode).CST Inputs.Torque actual value  sig_offset=616  sig_type=int16  type_size=16  sig_dim=1  device_id=0  sample_time=0.004000
      settings: SourceProductBaseCode=XP
  EtherCAT PDO Receive1 : xpcethercatlib/EtherCAT PDO Receive  Priority=2  sig_name=M2.Module 1 (CST Mode).CST Inputs.Torque actual value  sig_offset=792  sig_type=int16  type_size=16  sig_dim=1  device_id=0  sample_time=0.004000
      settings: SourceProductBaseCode=XP
  Mtorque : DataTypeConversion  OutDataTypeStr=double
  Mtorque1 : DataTypeConversion  OutDataTypeStr=double
  Side Torques : Gain  Gain=-1
  Side Torques1 : Gain  Gain=-1
  Torque Mapping : Gain  Gain=(3.6*104.92)/1000
  Torque Mapping1 : Gain  Gain=(3.6*104.92)/1000
  capstan reduction : Gain  Gain=5
  capstan reduction1 : Gain  Gain=5
  Side Torque : Outport
  wires:
  EtherCAT PDO Receive/1 -> Mtorque/1  "M1 Torque"
  Torque Mapping/1 -> capstan reduction/1
  Mtorque/1 -> Torque Mapping/1  "Motor Torque"
  EtherCAT PDO Receive1/1 -> Mtorque1/1  "M2 Torque"
  capstan reduction/1 -> Side Torques/1
  capstan reduction1/1 -> Side Torques1/1
  Torque Mapping1/1 -> capstan reduction1/1
  Side Torques1/1 -> Bus Creator/2  "M2 Side Torques"
  Mtorque1/1 -> Torque Mapping1/1  "Motor Torque"
  Bus Creator/1 -> Side Torque/1
  Side Torques/1 -> Bus Creator/1  "M1 Side Torques"

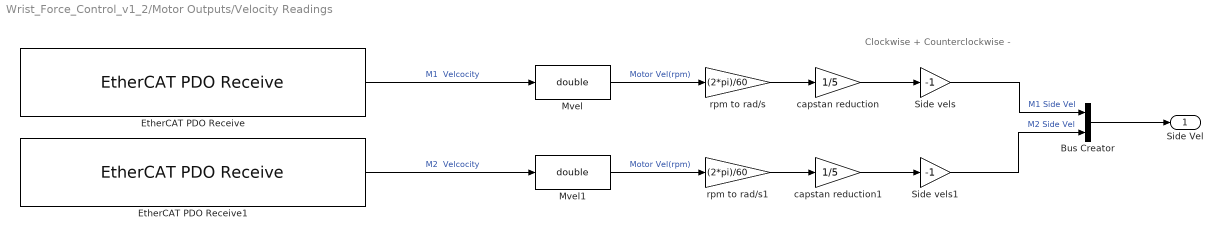
== system Wrist_Force_Control_v1_2/Motor Outputs/Velocity Readings ==
  note: Clockwise + Counterclockwise -
  Bus Creator : BusCreator  Inputs=2
  EtherCAT PDO Receive : xpcethercatlib/EtherCAT PDO Receive  Priority=2  sig_name=M1.Module 1 (CST Mode).CST Inputs.Velocity actual value averaged  sig_offset=632  sig_type=int32  type_size=32  sig_dim=1  device_id=0  sample_time=0.004000
      settings: SourceProductBaseCode=XP
  EtherCAT PDO Receive1 : xpcethercatlib/EtherCAT PDO Receive  Priority=2  sig_name=M2.Module 1 (CST Mode).CST Inputs.Velocity actual value averaged  sig_offset=760  sig_type=int32  type_size=32  sig_dim=1  device_id=0  sample_time=0.004000
      settings: SourceProductBaseCode=XP
  Mvel : DataTypeConversion  OutDataTypeStr=double
  Mvel1 : DataTypeConversion  OutDataTypeStr=double
  Side vels : Gain  Gain=-1
  Side vels1 : Gain  Gain=-1
  capstan reduction : Gain  Gain=1/5
  capstan reduction1 : Gain  Gain=1/5
  rpm to rad/s : Gain  Gain=(2*pi)/60
  rpm to rad/s1 : Gain  Gain=(2*pi)/60
  Side Vel : Outport
  wires:
  capstan reduction/1 -> Side vels/1
  EtherCAT PDO Receive1/1 -> Mvel1/1  "M2  Velcocity"
  Mvel/1 -> rpm to rad/s/1  "Motor Vel(rpm)"
  rpm to rad/s/1 -> capstan reduction/1
  EtherCAT PDO Receive/1 -> Mvel/1  "M1  Velcocity"
  rpm to rad/s1/1 -> capstan reduction1/1
  Mvel1/1 -> rpm to rad/s1/1  "Motor Vel(rpm)"
  capstan reduction1/1 -> Side vels1/1
  Side vels/1 -> Bus Creator/1  "M1 Side Vel"
  Bus Creator/1 -> Side Vel/1
  Side vels1/1 -> Bus Creator/2  "M2 Side Vel"

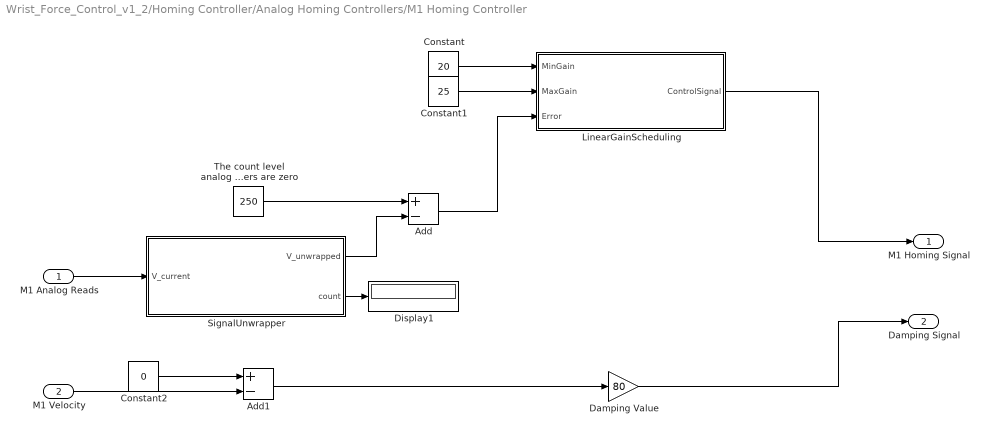
== system Wrist_Force_Control_v1_2/Homing Controller/Analog Homing Controllers/M1 Homing Controller ==
  M1 Analog Reads : Inport
  M1 Velocity : Inport  Port=2
  Add : Sum  Inputs=+-
  Add1 : Sum  Inputs=+-
  Constant : Constant  Value=20
  Constant1 : Constant  Value=25
  Constant2 : Constant  Value=0
  Damping Value : Gain  Gain=80
  Display1 : Display
  LinearGainScheduling : MATLAB Function  TreatAsAtomicUnit=on
  SignalUnwrapper : MATLAB Function  TreatAsAtomicUnit=on
  The count level analog encoders are zero : Constant  Value=250
  M1 Homing Signal : Outport
  Damping Signal : Outport  Port=2
  wires:
  SignalUnwrapper/1(V_unwrapped) -> Add/2
  The count level analog encoders are zero/1 -> Add/1
  M1 Analog Reads/1 -> SignalUnwrapper/1(V_current)
  Constant/1 -> LinearGainScheduling/1(MinGain)
  Constant1/1 -> LinearGainScheduling/2(MaxGain)
  SignalUnwrapper/2(count) -> Display1/1
  Add1/1 -> Damping Value/1
  M1 Velocity/1 -> Add1/2
  Add/1 -> LinearGainScheduling/3(Error)
  Constant2/1 -> Add1/1
  Damping Value/1 -> Damping Signal/1
  LinearGainScheduling/1(ControlSignal) -> M1 Homing Signal/1

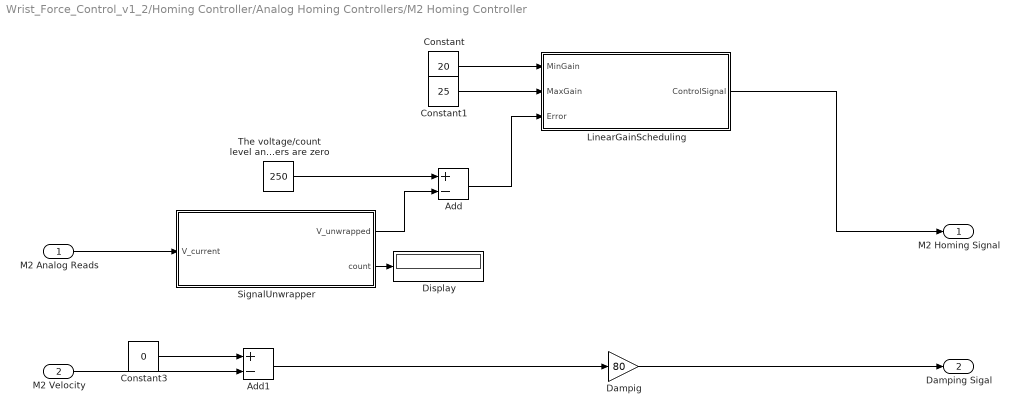
== system Wrist_Force_Control_v1_2/Homing Controller/Analog Homing Controllers/M2 Homing Controller ==
  M2 Analog Reads : Inport
  M2 Velocity : Inport  Port=2
  Add : Sum  Inputs=+-
  Add1 : Sum  Inputs=+-
  Constant : Constant  Value=20
  Constant1 : Constant  Value=25
  Constant3 : Constant  Value=0
  Dampig : Gain  Gain=80
  Display : Display
  LinearGainScheduling : MATLAB Function  TreatAsAtomicUnit=on
  SignalUnwrapper : MATLAB Function  TreatAsAtomicUnit=on
  The voltage/count level analog encoders are zero : Constant  Value=250
  M2 Homing Signal : Outport
  Damping Sigal : Outport  Port=2
  wires:
  SignalUnwrapper/2(count) -> Display/1
  M2 Analog Reads/1 -> SignalUnwrapper/1(V_current)
  LinearGainScheduling/1(ControlSignal) -> M2 Homing Signal/1
  The voltage/count level analog encoders are zero/1 -> Add/1
  SignalUnwrapper/1(V_unwrapped) -> Add/2
  Add/1 -> LinearGainScheduling/3(Error)
  Constant/1 -> LinearGainScheduling/1(MinGain)
  Constant1/1 -> LinearGainScheduling/2(MaxGain)
  Add1/1 -> Dampig/1
  M2 Velocity/1 -> Add1/2
  Constant3/1 -> Add1/1
  Dampig/1 -> Damping Sigal/1

== system Wrist_Force_Control_v1_2/Motor Inputs/Torque Mappig and Saturation /Torque Saturation ==
  demanded torque : Inport
  Demux : Demux  Outputs=2
  Mux1 : Mux  Inputs=2
  Saturation Dynamic : simulink/Discontinuities/Saturation Dynamic  OutMin=[]  OutMax=[]  OutDataTypeStr=Inherit: Same as second input  OutDataType=fixdt(1, 16)  OutScaling=2^-10  RndMeth=Simplest  DoSatur=off
  Saturation Dynamic1 : simulink/Discontinuities/Saturation Dynamic  OutMin=[]  OutMax=[]  OutDataTypeStr=Inherit: Same as second input  OutDataType=fixdt(1, 16)  OutScaling=2^-10  RndMeth=Simplest  DoSatur=off
  Torque Limit : DataStoreRead  DataStoreName=Motor_torque_limit
  negative : Gain  Gain=-1  OutDataTypeStr=double
  adjusted torque : Outport
  wires:
  Torque Limit/1 -> Saturation Dynamic/1, Saturation Dynamic1/1, negative/1
  Demux/2 -> Saturation Dynamic1/2
  Demux/1 -> Saturation Dynamic/2
  Mux1/1 -> adjusted torque/1
  negative/1 -> Saturation Dynamic/3, Saturation Dynamic1/3
  Saturation Dynamic1/1 -> Mux1/2
  Saturation Dynamic/1 -> Mux1/1
  demanded torque/1 -> Demux/1

== matlab function Wrist_Force_Control_v1_2/Subsystem/Forward Kinematics ==
  data: Motor1_Position input; pitch output; Motor2_Position input; roll output
function [pitch,roll] = Forward_Kinematics_Wrist(Motor1_Position, Motor2_Position)
% N = 5; % Capstan Ratio
d = 25; % mm 
D = 25; %mm 
pitch = (Motor1_Position + Motor2_Position)/2;
roll = ((Motor1_Position - Motor2_Position)/(2))*(d/D);

== matlab function Wrist_Force_Control_v1_2/Jacobian Transpose ==
  data: PitchTorqueContolSignal input; Motor1ForceInput output; RollControlSignal input; Motor2ForceInput output
function [Motor1ForceInput,Motor2ForceInput] = Jacobian_Transpose(PitchTorqueContolSignal, RollControlSignal)
N = 5; % Capstan Ratio
d = 25; % mm 
D = 25; %mm 
% Define the Jacobian Transpose
J_T = [1/(2*N),  d/(2*N*D);
       1/(2*N), -d/(2*N*D)];
% End-effector velocity vector
TorqueControlSignals = [PitchTorqueContolSignal; RollControlSignal];
% Compute the motor velocities
MotorForceInputs = J_T * TorqueControlSignals;
% Extract outputs
Motor1ForceInput = MotorForceInputs(1);
Motor2ForceInput = MotorForceInputs(2);

== matlab function Wrist_Force_Control_v1_2/Subsystem/Jacobian ==
  data: Motor1_velocity input; phi_dot output; Motor2_Velocity input; gamma_dot output
function [phi_dot, gamma_dot] = Jacobian_Wrist(Motor1_velocity, Motor2_Velocity)
 
N = 5; % Capstan Ratio
d = 25; % mm 
D = 25; %mm 
% Define the Jacobian matrix
J = [1/(2*N),  1/(2*N);
d/(2*N*D), -d/(2*N*D)];
% Motor velocity vector
theta_dot = [Motor1_velocity; Motor2_Velocity];
% Compute the end-effector velocities
x_dot = J * theta_dot;
% Extract outputs
phi_dot = x_dot(1);
gamma_dot = x_dot(2);

== matlab function Wrist_Force_Control_v1_2/Subsystem/MATLAB Function ==
  data: M1_Torque input; Pitch_Torque output; M2_Torque input; Roll_Torque output
function [Pitch_Torque,Roll_Torque]= ForwardDyamic(M1_Torque, M2_Torque)

Pitch_Torque = M1_Torque + M2_Torque;
Roll_Torque = M1_Torque - M2_Torque;

== matlab function Wrist_Force_Control_v1_2/Homing Controller/Analog Homing Controllers/M2 Homing Controller/SignalUnwrapper ==
  data: V_current input; V_unwrapped output; count output
function [V_unwrapped,count]= ScaledAnalogUnwrapper(V_current)
    % Scaled analog encoder input: 0-50 instead of 0-5 V
    % Persistent variables to store previous voltage and rotation count
    persistent V_prev rot_count
    
    if isempty(V_prev)
        V_prev = V_current;
        rot_count = 0;
    end
    % Calculate difference between current and previous
    delta = V_current - V_prev;
    % Threshold is 25 due to scaling (half of 50)
    if delta > 280
        rot_count = rot_count - 1;  % wrapped backward
    elseif delta < -220
        rot_count = rot_count + 1;  % wrapped forward
    end
    V_prev = V_current;
    count = rot_count;
    % Unwrap the signal (each rotation adds/subtracts 50 units)
    V_unwrapped = V_current + 50 * rot_count;
    
end

== matlab function Wrist_Force_Control_v1_2/Homing Controller/Analog Homing Controllers/M1 Homing Controller/LinearGainScheduling ==
  data: MinGain input; ControlSignal output; MaxGain input; Error input
function ControlSignal = LinearGainScheduling(MinGain, MaxGain, Error)
%IMPORTANT: Adjust according to workspace limits
MaxError = 300; 
if Error > MaxError
   MaxError = Error;
end
Gain = MinGain + (MaxGain - MinGain) * (abs(Error)/MaxError);
ControlSignal = Error*Gain;

== matlab function Wrist_Force_Control_v1_2/Homing Controller/Analog Homing Controllers/M1 Homing Controller/SignalUnwrapper ==
  data: V_current input; V_unwrapped output; count output
function [V_unwrapped,count] = ScaledAnalogUnwrapper(V_current)
    % Unwrapps the voltage levels to prevent error jumps
    % Persistent variables to store previous voltage and rotation count
    persistent V_prev rot_count
    
    if isempty(V_prev)
        V_prev = V_current;
        rot_count = 0;
    end
    % Calculate difference between current and previous
    delta = V_current - V_prev;
    % Threshold is 25 due to scaling (half of 50)
    if delta > 280
        rot_count = rot_count - 1;  % wrapped backward
    elseif delta < -220
        rot_count = rot_count + 1;  % wrapped forward
    end
    V_prev = V_current;
    count = rot_count;
    % Unwrap the signal (each rotation adds/subtracts 50 units)
    V_unwrapped = V_current + 50 * rot_count;
    
end

== matlab function Wrist_Force_Control_v1_2/Homing Controller/Analog Homing Controllers/M2 Homing Controller/LinearGainScheduling ==
  data: MinGain input; ControlSignal output; MaxGain input; Error input
function ControlSignal  = LinearGainScheduling(MinGain, MaxGain, Error)
%IMPORTANT: Adjust according to workspace limits
MaxError = 300; 
if Error > MaxError
   MaxError = Error;
end
Gain = MinGain + (MaxGain - MinGain) * (abs(Error)/MaxError);
ControlSignal = Error*Gain;
